simulink model "Control4GDL"  (R2024b)
settings: Solver=VariableStepAuto  StartTime=0.0  StopTime=6  RelTol=1e-3
settings Model: Creator=SNGULAR  LastModifiedBy=SNGULAR

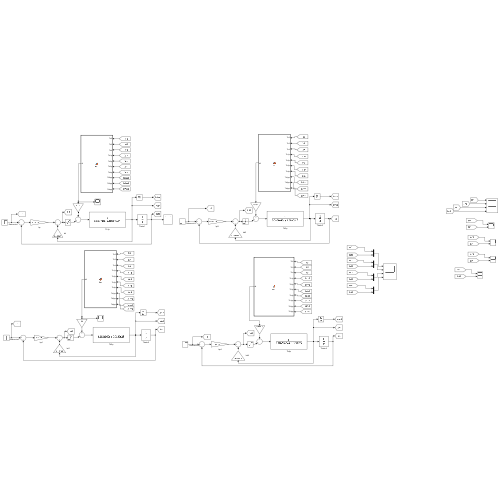
[thumbnail: Simulink's stored preview of the top-level diagram]
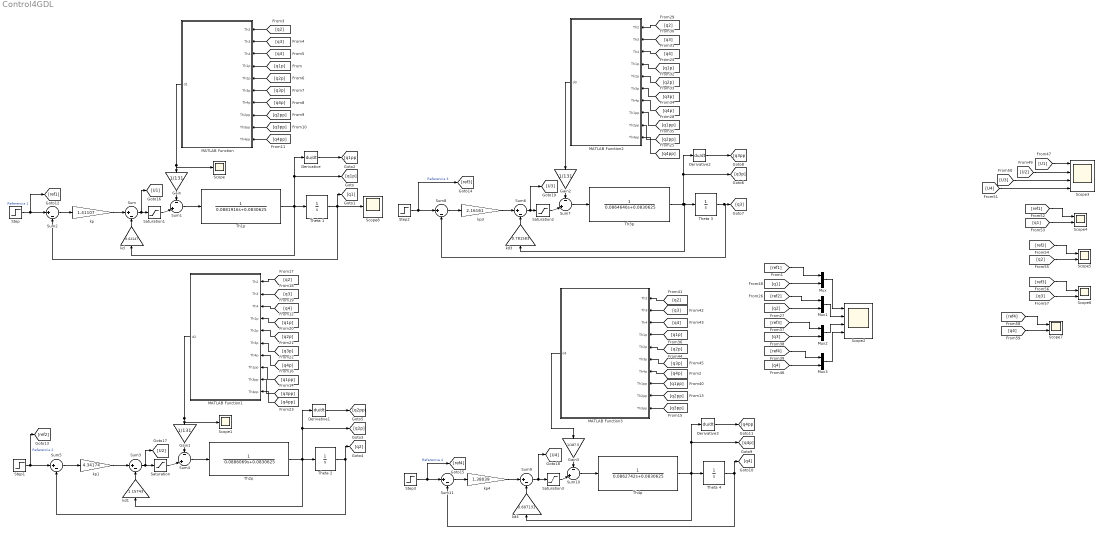
== system Control4GDL ==
  Derivative{,1..3} (4 alike) : Derivative
  Gain : Gain  Gain=1/131
  Gain1 : Gain  Gain=1/131
  Gain2 : Gain  Gain=1/131
  Gain3 : Gain  Gain=1/187.5
  MATLAB Function : MATLAB Function  TreatAsAtomicUnit=on
  MATLAB Function1 : MATLAB Function  TreatAsAtomicUnit=on
  MATLAB Function2 : MATLAB Function  TreatAsAtomicUnit=on
  MATLAB Function3 : MATLAB Function  TreatAsAtomicUnit=on
  Mux{,1..3} (4 alike) : Mux  Inputs=2
  Saturation{,1..3} (4 alike) : Saturate  UpperLimit=12  LowerLimit=-12
  Scope : Scope
  Scope1 : Scope
  Scope2 : Scope  NumInputPorts=4
  Scope3 : Scope  NumInputPorts=4
  Scope{4..7} (4 alike) : Scope  NumInputPorts=2
  Scope8 : Scope
  Step : Step  Time=0  After=pi/2  SampleTime=0
  Step1 : Step  Time=0  After=0  SampleTime=0
  Step2 : Step  Time=0  After=0  SampleTime=0
  Step3 : Step  Time=0  After=pi/3  SampleTime=0
  Sum{,2..3,5..6,8..9,11} (8 alike) : Sum  Inputs=|+-
  Sum{1,4,7,10} (4 alike) : Sum  Inputs=-|+|
  Th1p : TransferFcn  Denominator=[0.0881916 0.0830625]
  Th2p : TransferFcn  Denominator=[0.0886069 0.0830625]
  Th3p : TransferFcn  Denominator=[0.0864646 0.0830625]
  Th4p : TransferFcn  Denominator=[0.0862742 0.0830625]
  Theta {1..4} (4 alike) : Integrator
  kd : Gain  Gain=0.62247
  kd1 : Gain  Gain=1.15743
  kd3 : Gain  Gain=0.781583
  kd4 : Gain  Gain=0.607131
  kp : Gain  Gain=1.41107
  kp1 : Gain  Gain=4.34174
  kp3 : Gain  Gain=2.16161
  kp4 : Gain  Gain=1.38039
  wires:
  Th1p/1 -> kd/1, Derivative/1, [q1p], Theta 1/1
  Theta 1/1 -> [q1], Scope8/1, Sum2/2
  Sum2/1 -> kp/1
  kp/1 -> Sum/1
  kd/1 -> Sum/2
  Gain/1 -> Sum1/1
  Sum1/1 -> Th1p/1
  MATLAB Function/1(d1) -> Scope/1, Gain/1
  Derivative/1 -> [q1pp]
  [q1p] -> MATLAB Function/4(Th1p)
  [q2] -> MATLAB Function/1(Th2)
  [q3] -> MATLAB Function/2(Th3)
  [q4] -> MATLAB Function/3(Th4)
  [q2p] -> MATLAB Function/5(Th2p)
  [q3p] -> MATLAB Function/6(Th3p)
  [q4p] -> MATLAB Function/7(Th4p)
  [q2pp] -> MATLAB Function/8(Th2pp)
  [q3pp] -> MATLAB Function/9(Th3pp)
  [q4pp] -> MATLAB Function/10(Th4pp)
  Step/1 -> Sum2/1, [ref1]  "Referencia 1"
  Step1/1 -> [ref2], Sum5/1  "Referencia 2"
  [q3pp] -> MATLAB Function1/9(Th3pp)
  [q4p] -> MATLAB Function1/7(Th4p)
  [q3p] -> MATLAB Function1/6(Th3p)
  [q2p] -> MATLAB Function1/5(Th2p)
  [q4] -> MATLAB Function1/3(Th4)
  [q3] -> MATLAB Function1/2(Th3)
  [q2] -> MATLAB Function1/1(Th2)
  [q1pp] -> MATLAB Function1/8(Th1pp)
  [q1p] -> MATLAB Function1/4(Th1p)
  Derivative1/1 -> [q2pp]
  MATLAB Function1/1(d2) -> Scope1/1, Gain1/1
  Sum4/1 -> Th2p/1
  Gain1/1 -> Sum4/1
  kd1/1 -> Sum3/2
  Theta 2/1 -> Sum5/2, [q2]
  Th2p/1 -> Theta 2/1, [q2p], Derivative1/1, kd1/1
  Th3p/1 -> Derivative2/1, [q3p], kd3/1, Theta 3/1
  Theta 3/1 -> Sum8/2, [q3]
  Sum8/1 -> kp3/1
  kp3/1 -> Sum6/1
  Gain2/1 -> Sum7/1
  Sum7/1 -> Th3p/1
  MATLAB Function2/1(d3) -> Gain2/1
  Derivative2/1 -> [q3pp]
  [q1p] -> MATLAB Function2/4(Th1p)
  [q1pp] -> MATLAB Function2/8(Th1pp)
  [q2] -> MATLAB Function2/1(Th2)
  [q3] -> MATLAB Function2/2(Th3)
  [q4] -> MATLAB Function2/3(Th4)
  [q2p] -> MATLAB Function2/5(Th2p)
  [q3p] -> MATLAB Function2/6(Th3p)
  [q4p] -> MATLAB Function2/7(Th4p)
  [q2pp] -> MATLAB Function2/9(Th2pp)
  Step2/1 -> [ref3], Sum8/1  "Referencia 3"
  Step3/1 -> [ref4], Sum11/1  "Referencia 4"
  [q3p] -> MATLAB Function3/6(Th3p)
  [q2p] -> MATLAB Function3/5(Th2p)
  [q4] -> MATLAB Function3/3(Th4)
  [q3] -> MATLAB Function3/2(Th3)
  [q2] -> MATLAB Function3/1(Th2)
  [q1pp] -> MATLAB Function3/8(Th1pp)
  [q1p] -> MATLAB Function3/4(Th1p)
  Derivative3/1 -> [q4pp]
  MATLAB Function3/1(d4) -> Gain3/1
  Sum10/1 -> Th4p/1
  Gain3/1 -> Sum10/1
  kd4/1 -> Sum9/2
  kp4/1 -> Sum9/1
  Sum11/1 -> kp4/1
  Theta 4/1 -> Sum11/2, [q4]
  Th4p/1 -> Theta 4/1, [q4p], Derivative3/1, kd4/1
  [q1] -> Mux/2
  [ref1] -> Mux/1
  [q4p] -> MATLAB Function3/7(Th4p)
  [q2pp] -> MATLAB Function3/9(Th2pp)
  [q3pp] -> MATLAB Function3/10(Th3pp)
  [q4pp] -> MATLAB Function1/10(Th4pp)
  [q4pp] -> MATLAB Function2/10(Th4pp)
  Mux/1 -> Scope2/1
  [ref2] -> Mux1/1
  [q2] -> Mux1/2
  [q3] -> Mux2/2
  [ref3] -> Mux2/1
  [ref4] -> Mux3/1
  [q4] -> Mux3/2
  Mux1/1 -> Scope2/2
  Mux2/1 -> Scope2/3
  Mux3/1 -> Scope2/4
  Sum3/1 -> [U2], Saturation/1
  Saturation/1 -> Sum4/2
  Sum/1 -> [U1], Saturation1/1
  Saturation1/1 -> Sum1/2
  Sum6/1 -> [U3], Saturation2/1
  Saturation2/1 -> Sum7/2
  Sum9/1 -> [U4], Saturation3/1
  Saturation3/1 -> Sum10/2
  [U1] -> Scope3/1
  [U2] -> Scope3/2
  [U3] -> Scope3/3
  [U4] -> Scope3/4
  kp1/1 -> Sum3/1
  Sum5/1 -> kp1/1
  [ref2] -> Scope5/1
  [q2] -> Scope5/2
  [q1] -> Scope4/2
  [ref1] -> Scope4/1
  kd3/1 -> Sum6/2
  [q3] -> Scope6/2
  [ref3] -> Scope6/1
  [ref4] -> Scope7/1
  [q4] -> Scope7/2

== matlab function Control4GDL/MATLAB Function1 ==
  data: Th2 input; Th3 input; Th4 input; d2 output; Th1p input; Th2p input; Th3p input; Th4p input; Th1pp input; Th3pp input; Th4pp input
function d2 = fcn(Th2, Th3, Th4, Th1p, Th2p, Th3p, Th4p, Th1pp,Th3pp,Th4pp)

%% -------------------------------------------------------------
%  Parámetros del robot (desde tabla)
%  Todas las inercias convertidas de g·mm² -> kg·m² (×1e-9)
% --------------------------------------------------------------
%% MASAS
M1 = 0.14628;     % [kg]
M2 = 0.14239;     % [kg]
M3 = 0.17884;     % [kg]

%% GRAVEDAD
grav = 9.81;      % [m/s^2]

%% INERCIAS DEL ESLABÓN 1 (g·mm² → kg·m²)
I1xx = 237354.33 * 1e-9;
I1xy = 0          * 1e-9;
I1xz = 0          * 1e-9;

I1yx = 0          * 1e-9;
I1yy = 294106.43  * 1e-9;
I1yz = -200.13    * 1e-9;

I1zx = 0          * 1e-9;
I1zy = -200.13    * 1e-9;
I1zz = 126421.47  * 1e-9;

%% INERCIAS DEL ESLABÓN 2
I2xx = 316936.55  * 1e-9;
I2xy = 0          * 1e-9;
I2xz = -697.68    * 1e-9;

I2yx = 0          * 1e-9;
I2yy = 507105.45  * 1e-9;
I2yz = 0          * 1e-9;

I2zx = -697.68    * 1e-9;
I2zy = 0          * 1e-9;
I2zz = 231758.79  * 1e-9;

%% INERCIAS DEL ESLABÓN 3
I3xx = 588562.90  * 1e-9;
I3xy = 0          * 1e-9;
I3xz = 0          * 1e-9;

I3yx = 0          * 1e-9;
I3yy = 158273.82  * 1e-9;
I3yz = 12715.89   * 1e-9;

I3zx = 0          * 1e-9;
I3zy = 12715.89   * 1e-9;
I3zz = 469157.76  * 1e-9;

%% DISTANCIAS Y LONGITUDES
d1    = 0.046;    % [m]
d1cm  = 0.023;    % [m]

a2    = 0.08550;  % [m]
a2cm  = 0.04275;  % [m]

d4    = 0.080;    % [m]
d4cm  = 0.040;    % [m]



%% Cálculo de d2
d2=(1/2).*(2.*a2cm.*grav.*M2.*cos(Th2)+2.*I2zy.*Th1pp.*cos(Th2)+2.* ...
d4cm.*M3.*Th3pp.*(d4cm+a2.*cos(Th3))+2.*grav.*M3.*(a2.*cos(Th2)+ ...
d4cm.*cos(Th2+Th3))+2.*I2zx.*Th1pp.*sin(Th2)+(-4).*a2.*d4cm.*M3.* ...
Th2p.*Th3p.*sin(Th3)+(-2).*a2.*d4cm.*M3.*Th3p.^2.*sin(Th3)+2.* ...
Th4pp.*(I3yz.*cos(Th4)+I3xz.*sin(Th4))+2.*Th1pp.*sin(Th2+Th3).*( ...
I3yz.*cos(Th4)+I3xz.*sin(Th4))+2.*Th4p.^2.*(I3xz.*cos(Th4)+(-1).* ...
I3yz.*sin(Th4))+Th1p.*Th3p.*((I3xy+(-1).*I3yx).*sin(Th2+Th3)+cos( ...
Th2+Th3).*((I3yz+(-1).*I3zy).*cos(Th4)+(I3xz+(-1).*I3zx).*sin(Th4) ...
))+(-1).*Th1p.*Th2p.*((I2xz+(-1).*I2zx).*cos(Th2)+((-1).*I2yz+ ...
I2zy).*sin(Th2)+((-1).*I3xy+I3yx).*sin(Th2+Th3)+cos(Th2+Th3).*((( ...
-1).*I3yz+I3zy).*cos(Th4)+((-1).*I3xz+I3zx).*sin(Th4)))+Th3pp.*( ...
I3xx+I3yy+((-1).*I3xx+I3yy).*cos(2.*Th4)+(I3xy+I3yx).*sin(2.*Th4)) ...
+Th1pp.*cos(Th2+Th3).*((-1).*I3xy+I3yx+(I3xy+I3yx).*cos(2.*Th4)+( ...
I3xx+(-1).*I3yy).*sin(2.*Th4))+Th2p.*Th4p.*(2.*(I3xy+I3yx).*cos( ...
2.*Th4)+2.*(I3xx+(-1).*I3yy).*sin(2.*Th4))+Th3p.*Th4p.*(2.*(I3xy+ ...
I3yx).*cos(2.*Th4)+2.*(I3xx+(-1).*I3yy).*sin(2.*Th4))+(1/2).* ...
Th1p.^2.*((-2).*(I2xy+I2yx).*cos(2.*Th2)+2.*((-1).*I2xx+I2yy).* ...
sin(2.*Th2)+2.*a2cm.^2.*M2.*sin(2.*Th2)+2.*M3.*(a2.^2.*sin(2.*Th2) ...
+d4cm.^2.*sin(2.*(Th2+Th3))+2.*a2.*d4cm.*sin(2.*Th2+Th3))+2.*cos( ...
2.*(Th2+Th3)).*((-1).*(I3xz+I3zx).*cos(Th4)+(I3yz+I3zy).*sin(Th4)) ...
+sin(2.*(Th2+Th3)).*(I3xx+I3yy+(-2).*I3zz+(I3xx+(-1).*I3yy).*cos( ...
2.*Th4)+(-1).*(I3xy+I3yx).*sin(2.*Th4)))+Th1p.*Th4p.*(2.*sin(Th2+ ...
Th3).*(I3xz.*cos(Th4)+(-1).*I3yz.*sin(Th4))+(-1).*cos(Th2+Th3).*( ...
I3zz+((-1).*I3xx+I3yy).*cos(2.*Th4)+(I3xy+I3yx).*sin(2.*Th4)))+ ...
Th1p.*Th4p.*(sin(Th2+Th3).*((I3xz+I3zx).*cos(Th4)+(-1).*(I3yz+ ...
I3zy).*sin(Th4))+(-1).*cos(Th2+Th3).*(I3zz+((-1).*I3xx+I3yy).*cos( ...
2.*Th4)+(I3xy+I3yx).*sin(2.*Th4))));

end

== matlab function Control4GDL/MATLAB Function ==
  data: Th2 input; Th3 input; Th4 input; d1 output; Th1p input; Th2p input; Th3p input; Th4p input; Th2pp input; Th3pp input; Th4pp input
function d1 = fcn( Th2, Th3, Th4, Th1p, Th2p, Th3p, Th4p, Th2pp, Th3pp, Th4pp )
%% -------------------------------------------------------------
%  Parámetros del robot (desde tabla)
%  Todas las inercias convertidas de g·mm² -> kg·m² (×1e-9)
% --------------------------------------------------------------

%% MASAS
M1 = 0.14628;     % [kg]
M2 = 0.14239;     % [kg]
M3 = 0.17884;     % [kg]

%% GRAVEDAD
grav = 9.81;      % [m/s^2]

%% INERCIAS DEL ESLABÓN 1 (g·mm² → kg·m²)
I1xx = 237354.33 * 1e-9;
I1xy = 0          * 1e-9;
I1xz = 0          * 1e-9;

I1yx = 0          * 1e-9;
I1yy = 294106.43  * 1e-9;
I1yz = -200.13    * 1e-9;

I1zx = 0          * 1e-9;
I1zy = -200.13    * 1e-9;
I1zz = 126421.47  * 1e-9;

%% INERCIAS DEL ESLABÓN 2
I2xx = 316936.55  * 1e-9;
I2xy = 0          * 1e-9;
I2xz = -697.68    * 1e-9;

I2yx = 0          * 1e-9;
I2yy = 507105.45  * 1e-9;
I2yz = 0          * 1e-9;

I2zx = -697.68    * 1e-9;
I2zy = 0          * 1e-9;
I2zz = 231758.79  * 1e-9;

%% INERCIAS DEL ESLABÓN 3
I3xx = 588562.90  * 1e-9;
I3xy = 0          * 1e-9;
I3xz = 0          * 1e-9;

I3yx = 0          * 1e-9;
I3yy = 158273.82  * 1e-9;
I3yz = 12715.89   * 1e-9;

I3zx = 0          * 1e-9;
I3zy = 12715.89   * 1e-9;
I3zz = 469157.76  * 1e-9;

%% DISTANCIAS Y LONGITUDES
d1    = 0.046;    % [m]
d1cm  = 0.023;    % [m]

a2    = 0.08550;  % [m]
a2cm  = 0.04275;  % [m]

d4    = 0.080;    % [m]
d4cm  = 0.040;    % [m]


%% -------------------------------------------------------------
%   Cálculo de d1 
% -------------------------------------------------------------
d1 =(1/2).*(2.*I2yz.*Th2pp.*cos(Th2)+2.*I2xz.*Th2pp.*sin(Th2)+2.* ...
I3zz.*Th4pp.*sin(Th2+Th3)+(-2).*Th4p.^2.*cos(Th2+Th3).*(I3yz.*cos( ...
Th4)+I3xz.*sin(Th4))+2.*Th4pp.*cos(Th2+Th3).*(I3xz.*cos(Th4)+(-1) ...
.*I3yz.*sin(Th4))+2.*Th2pp.*sin(Th2+Th3).*(I3zy.*cos(Th4)+I3zx.* ...
sin(Th4))+2.*Th3pp.*sin(Th2+Th3).*(I3zy.*cos(Th4)+I3zx.*sin(Th4))+ ...
Th2pp.*cos(Th2+Th3).*(I3xy+(-1).*I3yx+(I3xy+I3yx).*cos(2.*Th4)+( ...
I3xx+(-1).*I3yy).*sin(2.*Th4))+Th3pp.*cos(Th2+Th3).*(I3xy+(-1).* ...
I3yx+(I3xy+I3yx).*cos(2.*Th4)+(I3xx+(-1).*I3yy).*sin(2.*Th4))+2.* ...
Th2p.*Th4p.*(sin(Th2+Th3).*(((-1).*I3xz+I3zx).*cos(Th4)+(I3yz+(-1) ...
.*I3zy).*sin(Th4))+cos(Th2+Th3).*(I3zz+(I3xx+(-1).*I3yy).*cos(2.* ...
Th4)+(-1).*(I3xy+I3yx).*sin(2.*Th4)))+2.*Th3p.*Th4p.*(sin(Th2+Th3) ...
.*(((-1).*I3xz+I3zx).*cos(Th4)+(I3yz+(-1).*I3zy).*sin(Th4))+cos( ...
Th2+Th3).*(I3zz+(I3xx+(-1).*I3yy).*cos(2.*Th4)+(-1).*(I3xy+I3yx).* ...
sin(2.*Th4)))+Th1p.*Th3p.*((-4).*d4cm.*M3.*(a2.*cos(Th2)+d4cm.* ...
cos(Th2+Th3)).*sin(Th2+Th3)+2.*cos(2.*(Th2+Th3)).*((I3xz+I3zx).* ...
cos(Th4)+(-1).*(I3yz+I3zy).*sin(Th4))+sin(2.*(Th2+Th3)).*((-1).* ...
I3xx+(-1).*I3yy+2.*I3zz+((-1).*I3xx+I3yy).*cos(2.*Th4)+(I3xy+I3yx) ...
.*sin(2.*Th4)))+Th1p.*Th2p.*(2.*(I2xy+I2yx).*cos(2.*Th2)+2.*(I2xx+ ...
(-1).*I2yy).*sin(2.*Th2)+(-2).*a2cm.^2.*M2.*sin(2.*Th2)+(-2).*M3.* ...
(a2.^2.*sin(2.*Th2)+d4cm.^2.*sin(2.*(Th2+Th3))+2.*a2.*d4cm.*sin( ...
2.*Th2+Th3))+2.*cos(2.*(Th2+Th3)).*((I3xz+I3zx).*cos(Th4)+(-1).*( ...
I3yz+I3zy).*sin(Th4))+sin(2.*(Th2+Th3)).*((-1).*I3xx+(-1).*I3yy+ ...
2.*I3zz+((-1).*I3xx+I3yy).*cos(2.*Th4)+(I3xy+I3yx).*sin(2.*Th4)))+ ...
(-1).*Th1p.*Th4p.*(sin(2.*(Th2+Th3)).*((I3yz+I3zy).*cos(Th4)+( ...
I3xz+I3zx).*sin(Th4))+2.*cos(Th2+Th3).^2.*((I3xy+I3yx).*cos(2.* ...
Th4)+(I3xx+(-1).*I3yy).*sin(2.*Th4)))+2.*Th2p.*Th3p.*(2.*cos(Th2+ ...
Th3).*(I3zy.*cos(Th4)+I3zx.*sin(Th4))+(-1).*sin(Th2+Th3).*(I3xy+( ...
-1).*I3yx+(I3xy+I3yx).*cos(2.*Th4)+(I3xx+(-1).*I3yy).*sin(2.*Th4)) ...
)+Th3p.^2.*(2.*cos(Th2+Th3).*(I3zy.*cos(Th4)+I3zx.*sin(Th4))+(-1) ...
.*sin(Th2+Th3).*(I3xy+(-1).*I3yx+(I3xy+I3yx).*cos(2.*Th4)+(I3xx+( ...
-1).*I3yy).*sin(2.*Th4)))+Th2p.^2.*(2.*I2xz.*cos(Th2)+(-2).*I2yz.* ...
sin(Th2)+2.*cos(Th2+Th3).*(I3zy.*cos(Th4)+I3zx.*sin(Th4))+(-1).* ...
sin(Th2+Th3).*(I3xy+(-1).*I3yx+(I3xy+I3yx).*cos(2.*Th4)+(I3xx+(-1) ...
.*I3yy).*sin(2.*Th4))));

end

== matlab function Control4GDL/MATLAB Function2 ==
  data: Th2 input; Th3 input; Th4 input; d3 output; Th1p input; Th2p input; Th3p input; Th4p input; Th1pp input; Th2pp input; Th4pp input
function d3 = fcn(Th2, Th3, Th4, Th1p, Th2p, Th3p, Th4p, Th1pp,Th2pp,Th4pp)

%% -------------------------------------------------------------
%  Parámetros del robot (desde tabla)
%  Todas las inercias convertidas de g·mm² -> kg·m² (×1e-9)
% --------------------------------------------------------------
%% MASAS
M1 = 0.14628;     % [kg]
M2 = 0.14239;     % [kg]
M3 = 0.17884;     % [kg]

%% GRAVEDAD
grav = 9.81;      % [m/s^2]

%% INERCIAS DEL ESLABÓN 1 (g·mm² → kg·m²)
I1xx = 237354.33 * 1e-9;
I1xy = 0          * 1e-9;
I1xz = 0          * 1e-9;

I1yx = 0          * 1e-9;
I1yy = 294106.43  * 1e-9;
I1yz = -200.13    * 1e-9;

I1zx = 0          * 1e-9;
I1zy = -200.13    * 1e-9;
I1zz = 126421.47  * 1e-9;

%% INERCIAS DEL ESLABÓN 2
I2xx = 316936.55  * 1e-9;
I2xy = 0          * 1e-9;
I2xz = -697.68    * 1e-9;

I2yx = 0          * 1e-9;
I2yy = 507105.45  * 1e-9;
I2yz = 0          * 1e-9;

I2zx = -697.68    * 1e-9;
I2zy = 0          * 1e-9;
I2zz = 231758.79  * 1e-9;

%% INERCIAS DEL ESLABÓN 3
I3xx = 588562.90  * 1e-9;
I3xy = 0          * 1e-9;
I3xz = 0          * 1e-9;

I3yx = 0          * 1e-9;
I3yy = 158273.82  * 1e-9;
I3yz = 12715.89   * 1e-9;

I3zx = 0          * 1e-9;
I3zy = 12715.89   * 1e-9;
I3zz = 469157.76  * 1e-9;

%% DISTANCIAS Y LONGITUDES
d1    = 0.046;    % [m]
d1cm  = 0.023;    % [m]

a2    = 0.08550;  % [m]
a2cm  = 0.04275;  % [m]

d4    = 0.080;    % [m]
d4cm  = 0.040;    % [m]


%% Cálculo de d3
d3=(1/4).*(2.*d4cm.*M3.*(2.*grav.*cos(Th2+Th3)+2.*a2.*(Th2pp.*cos( ...
Th3)+Th2p.^2.*sin(Th3)+Th1p.^2.*cos(Th2).*sin(Th2+Th3)))+2.* ...
d4cm.^2.*M3.*(2.*Th2pp+Th1p.^2.*sin(2.*(Th2+Th3)))+Th1p.^2.*(2.* ...
cos(2.*(Th2+Th3)).*((-1).*(I3xz+I3zx).*cos(Th4)+(I3yz+I3zy).*sin( ...
Th4))+sin(2.*(Th2+Th3)).*(I3xx+I3yy+(-2).*I3zz+(I3xx+(-1).*I3yy).* ...
cos(2.*Th4)+(-1).*(I3xy+I3yx).*sin(2.*Th4)))+2.*(I3xx.*Th2pp+ ...
I3yy.*Th2pp+2.*I3xz.*Th4p.^2.*cos(Th4)+(-1).*I3xx.*Th2pp.*cos(2.* ...
Th4)+I3yy.*Th2pp.*cos(2.*Th4)+Th1pp.*cos(Th2+Th3).*((-1).*I3xy+ ...
I3yx+(I3xy+I3yx).*cos(2.*Th4))+2.*I3yz.*Th1pp.*cos(Th4).*sin(Th2+ ...
Th3)+(-2).*I3yz.*Th4p.^2.*sin(Th4)+2.*I3xz.*Th1pp.*sin(Th2+Th3).* ...
sin(Th4)+2.*Th4pp.*(I3yz.*cos(Th4)+I3xz.*sin(Th4))+I3xy.*Th2pp.* ...
sin(2.*Th4)+I3yx.*Th2pp.*sin(2.*Th4)+I3xx.*Th1pp.*cos(Th2+Th3).* ...
sin(2.*Th4)+(-1).*I3yy.*Th1pp.*cos(Th2+Th3).*sin(2.*Th4)+2.*Th2p.* ...
Th4p.*((I3xy+I3yx).*cos(2.*Th4)+(I3xx+(-1).*I3yy).*sin(2.*Th4))+ ...
2.*Th3p.*Th4p.*((I3xy+I3yx).*cos(2.*Th4)+(I3xx+(-1).*I3yy).*sin( ...
2.*Th4)))+2.*Th1p.*((Th2p+Th3p).*((I3xy+(-1).*I3yx).*sin(Th2+Th3)+ ...
cos(Th2+Th3).*((I3yz+(-1).*I3zy).*cos(Th4)+(I3xz+(-1).*I3zx).*sin( ...
Th4)))+Th4p.*(sin(Th2+Th3).*((3.*I3xz+I3zx).*cos(Th4)+(-1).*(3.* ...
I3yz+I3zy).*sin(Th4))+(-2).*cos(Th2+Th3).*(I3zz+((-1).*I3xx+I3yy) ...
.*cos(2.*Th4)+(I3xy+I3yx).*sin(2.*Th4)))));
end

== matlab function Control4GDL/MATLAB Function3 ==
  data: Th2 input; Th3 input; Th4 input; d4 output; Th1p input; Th2p input; Th3p input; Th4p input; Th1pp input; Th2pp input; Th3pp input
function d4 = fcn(Th2, Th3, Th4, Th1p, Th2p, Th3p,Th4p,Th1pp,Th2pp,Th3pp)

%% -------------------------------------------------------------
%  Parámetros del robot (desde tabla)
%  Todas las inercias convertidas de g·mm² -> kg·m² (×1e-9)
% --------------------------------------------------------------
%% MASAS
M1 = 0.14628;     % [kg]
M2 = 0.14239;     % [kg]
M3 = 0.17884;     % [kg]

%% GRAVEDAD
grav = 9.81;      % [m/s^2]

%% INERCIAS DEL ESLABÓN 1 (g·mm² → kg·m²)
I1xx = 237354.33 * 1e-9;
I1xy = 0          * 1e-9;
I1xz = 0          * 1e-9;

I1yx = 0          * 1e-9;
I1yy = 294106.43  * 1e-9;
I1yz = -200.13    * 1e-9;

I1zx = 0          * 1e-9;
I1zy = -200.13    * 1e-9;
I1zz = 126421.47  * 1e-9;

%% INERCIAS DEL ESLABÓN 2
I2xx = 316936.55  * 1e-9;
I2xy = 0          * 1e-9;
I2xz = -697.68    * 1e-9;

I2yx = 0          * 1e-9;
I2yy = 507105.45  * 1e-9;
I2yz = 0          * 1e-9;

I2zx = -697.68    * 1e-9;
I2zy = 0          * 1e-9;
I2zz = 231758.79  * 1e-9;

%% INERCIAS DEL ESLABÓN 3
I3xx = 588562.90  * 1e-9;
I3xy = 0          * 1e-9;
I3xz = 0          * 1e-9;

I3yx = 0          * 1e-9;
I3yy = 158273.82  * 1e-9;
I3yz = 12715.89   * 1e-9;

I3zx = 0          * 1e-9;
I3zy = 12715.89   * 1e-9;
I3zz = 469157.76  * 1e-9;

%% DISTANCIAS Y LONGITUDES
d1    = 0.046;    % [m]
d1cm  = 0.023;    % [m]

a2    = 0.08550;  % [m]
a2cm  = 0.04275;  % [m]

d4    = 0.080;    % [m]
d4cm  = 0.040;    % [m]



%% Cálculo de d4
d4=(1/4).*(Th1p.^2.*(sin(2.*(Th2+Th3)).*((I3yz+I3zy).*cos(Th4)+(I3xz+ ...
I3zx).*sin(Th4))+2.*cos(Th2+Th3).^2.*((I3xy+I3yx).*cos(2.*Th4)+( ...
I3xx+(-1).*I3yy).*sin(2.*Th4)))+2.*Th1p.*(Th4p.*cos(Th2+Th3).*(( ...
I3yz+(-1).*I3zy).*cos(Th4)+(I3xz+(-1).*I3zx).*sin(Th4))+Th2p.*( ...
sin(Th2+Th3).*((-1).*(I3xz+3.*I3zx).*cos(Th4)+(I3yz+3.*I3zy).*sin( ...
Th4))+2.*cos(Th2+Th3).*(I3zz+((-1).*I3xx+I3yy).*cos(2.*Th4)+(I3xy+ ...
I3yx).*sin(2.*Th4)))+Th3p.*(sin(Th2+Th3).*((-1).*(I3xz+3.*I3zx).* ...
cos(Th4)+(I3yz+3.*I3zy).*sin(Th4))+2.*cos(Th2+Th3).*(I3zz+((-1).* ...
I3xx+I3yy).*cos(2.*Th4)+(I3xy+I3yx).*sin(2.*Th4))))+(-2).*(Th3p.* ...
Th4p.*((I3xz+(-1).*I3zx).*cos(Th4)+((-1).*I3yz+I3zy).*sin(Th4))+( ...
-2).*((Th2pp+Th3pp).*(I3zy.*cos(Th4)+I3zx.*sin(Th4))+Th1pp.*( ...
I3zz.*sin(Th2+Th3)+cos(Th2+Th3).*(I3zx.*cos(Th4)+(-1).*I3zy.*sin( ...
Th4))))+Th2p.^2.*((I3xy+I3yx).*cos(2.*Th4)+(I3xx+(-1).*I3yy).*sin( ...
2.*Th4))+Th3p.^2.*((I3xy+I3yx).*cos(2.*Th4)+(I3xx+(-1).*I3yy).* ...
sin(2.*Th4))+Th2p.*(Th4p.*((I3xz+(-1).*I3zx).*cos(Th4)+((-1).* ...
I3yz+I3zy).*sin(Th4))+2.*Th3p.*((I3xy+I3yx).*cos(2.*Th4)+(I3xx+( ...
-1).*I3yy).*sin(2.*Th4)))));


end
